simulink model "Tarea1"  (R2023b)
settings: Solver=VariableStepAuto  StartTime=0.0  StopTime=10  RelTol=1e-3
values from neighbouring files (symbols this model uses):
  a = 4.52    [plantafcn.m]
  Jl = 10    [plantafcn.m]
  Jm = 0.005    [plantafcn.m]
  Ka = 5    [plantafcn.m]
  Kb = 0.0706    [plantafcn.m]
  Ki = 10    [plantafcn.m]
  Ko = 50    [plantafcn.m]
  Kv = 10    [plantafcn.m]
  n = 1/100    (= 0.01)    [plantafcn.m]
  N = 1    [plantafcn.m]
  Ra = 10    [plantafcn.m]
undefined symbols (not defined in the file or in its folder): x3_ss
libraries: slpidlib x1
settings Model: Creator=juanj  LastModifiedBy=juanj

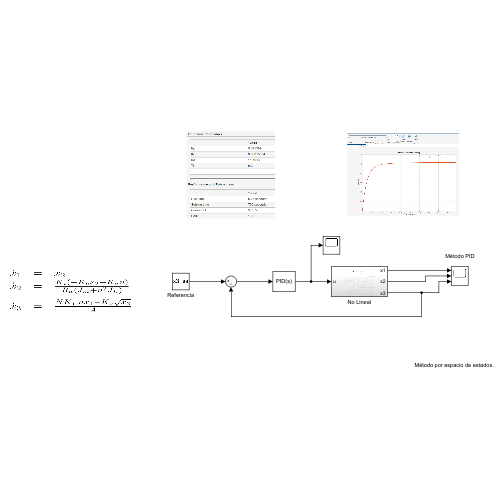
[thumbnail: Simulink's stored preview of the top-level diagram]
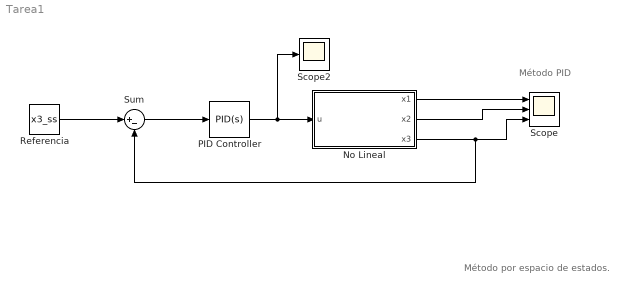
== system Tarea1 ==
  note: Método por espacio de estados.
  note: Método PID
  No Lineal : Subsystem
  PID Controller : slpidlib/PID Controller  Controller=PID  Form=Parallel  TimeDomain=Continuous-time  UseExternalTs=off  SampleTime=-1  IntegratorMethod=Forward Euler  FilterMethod=Forward Euler  ControllerParametersSource=internal  P=0.095359  I=0.00015684  UseKiTs=off  D=14.4946  N=100  UseFilter=on  TunerSelectOption=Transfer Function Based (PID Tuner App)  InitialConditionSource=internal  InitialConditionForIntegrator=0  InitialConditionForFilter=0  DifferentiatorICPrevScaledInput=0  ExternalReset=none  TrackingMode=off  Kt=1  LimitOutput=off  SatLimitsSource=internal  UpperSaturationLimit=inf  LowerSaturationLimit=-inf  LinearizeAsGain=on  AntiWindupMode=none  Kb=1  LimitIntegrator=off  UpperIntegratorSaturationLimit=inf  LowerIntegratorSaturationLimit=-inf  POutMin=[]  POutMax=[]  IOutMin=[]  IOutMax=[]  DOutMin=[]  DOutMax=[]  NOutMin=[]  NOutMax=[]  SumOutMin=[]  SumOutMax=[]  SaturationOutMin=[]  SaturationOutMax=[]  PParamMin=[]  PParamMax=[]  IParamMin=[]  IParamMax=[]  DParamMin=[]  DParamMax=[]  NParamMin=[]  NParamMax=[]  KbParamMin=[]  KbParamMax=[]  KtParamMin=[]  KtParamMax=[]  KbOutMin=[]  KbOutMax=[]  KtOutMin=[]  KtOutMax=[]  IntegratorOutMin=[]  IntegratorOutMax=[]  FilterOutMin=[]  FilterOutMax=[]  SumI1OutMin=[]  SumI1OutMax=[]  SumI2OutMin=[]  SumI2OutMax=[]  SumI3OutMin=[]  SumI3OutMax=[]  SumI4OutMin=[]  SumI4OutMax=[]  SumDOutMin=[]  SumDOutMax=[]  DifferentiatorOutMin=[]  DifferentiatorOutMax=[]  FilterDiffOutCoefMin=[]  FilterDiffOutCoefMax=[]  ReciprocalOutMin=[]  ReciprocalOutMax=[]  SumDenOutMin=[]  SumDenOutMax=[]  SumNumOutMin=[]  SumNumOutMax=[]  DivideOutMin=[]  DivideOutMax=[]  UdiffTsProdOutMin=[]  UdiffTsProdOutMax=[]  NTsProdOutMin=[]  NTsProdOutMax=[]  UintegralTsProdOutMin=[]  UintegralTsProdOutMax=[]  UngainTsProdOutMin=[]  UngainTsProdOutMax=[]  ClampingZeroOutDataTypeStr=Inherit: Inherit via back propagation  ClampingZeroOutMin=[]  ClampingZeroOutMax=[]  FilterDenConstantOutDataTypeStr=Inherit: Inherit via back propagation  FilterDenConstantOutMin=[]  FilterDenConstantOutMax=[]  PCopyOutDataTypeStr=Inherit: Inherit via back propagation  PCopyOutMin=[]  PCopyOutMax=[]  NCopyOutDataTypeStr=Inherit: Inherit via back propagation  NCopyOutMin=[]  NCopyOutMax=[]  IntegratorContinuousStateAttributes=''  IntegratorStateMustResolveToSignalObject=off  IntegratorRTWStateStorageClass=Auto  FilterContinuousStateAttributes=''  FilterStateMustResolveToSignalObject=off  FilterRTWStateStorageClass=Auto  ParallelPVariant=InternalParameters  IdealPVariant=Disabled  IVariant=InternalParameters  DVariant=InternalParameters  IntegratorVariant=Continuous  SatVariant=Disabled  AWVariant=Passthrough  PCopyVariant=Disabled  TRVariant=Disabled  FdbkBlocksVariant=Forward  IdealPFdbkVariant=Disabled  SatFdbkVariant=Disabled  DerivativeFilterVariant=ContFilter  NVariant=InternalParameters  NCopyVariant=Disabled  FilterICVariant=InternalICsFilter  IntegratorICVariant=InternalICs  ExternalResetVariant=Disabled  TRSumVariant=Passthrough  SumFdbkVariant=Disabled  SumVariant=Sum_PID  TsampFilterVariant=InternalTs  TsampNgainVariant=Passthrough  TsampIntegralVariant=Disabled_SignalSpec  ExternalSaturationOutDataTypeStr=Inherit: Same as second input
  Referencia : Constant  Value=x3_ss
  Scope : Scope  NumInputPorts=3
  Scope2 : Scope
  Sum : Sum  Inputs=|+-
  wires:
  Sum/1 -> PID Controller/1
  Referencia/1 -> Sum/1
  PID Controller/1 -> Scope2/1, No Lineal/1(u)
  No Lineal/3(x3) -> Sum/2, Scope/3
  No Lineal/1(x1) -> Scope/1
  No Lineal/2(x2) -> Scope/2

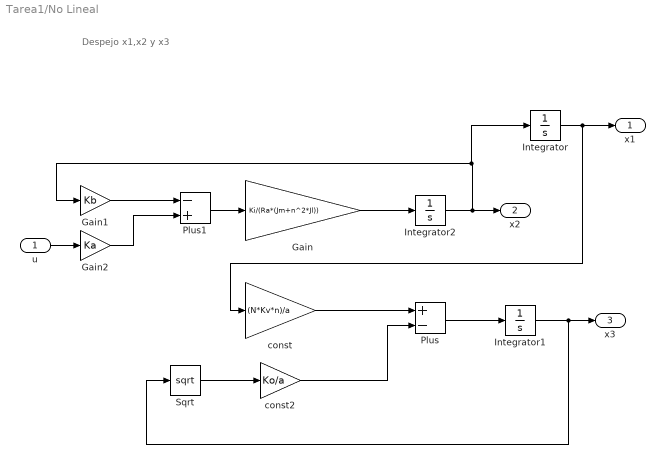
== system Tarea1/No Lineal ==
  note: Despejo x1,x2 y x3
  u : Inport
  Gain : Gain  Gain=Ki/(Ra*(Jm+n^2*Jl))
  Gain1 : Gain  Gain=Kb
  Gain2 : Gain  Gain=Ka
  Integrator : Integrator
  Integrator1 : Integrator
  Integrator2 : Integrator
  Plus : Sum  Inputs=+-
  Plus1 : Sum  Inputs=-+
  Sqrt : Sqrt
  const : Gain  Gain=(N*Kv*n)/a
  const2 : Gain  Gain=Ko/a
  x1 : Outport
  x2 : Outport  Port=2
  x3 : Outport  Port=3
  wires:
  Integrator/1 -> x1/1, const/1
  const/1 -> Plus/1
  const2/1 -> Plus/2
  Plus/1 -> Integrator1/1
  Sqrt/1 -> const2/1
  Integrator1/1 -> Sqrt/1, x3/1
  Gain/1 -> Integrator2/1
  Gain1/1 -> Plus1/1
  Gain2/1 -> Plus1/2
  Plus1/1 -> Gain/1
  Integrator2/1 -> Integrator/1, Gain1/1, x2/1
  u/1 -> Gain2/1
